simulink model "sampleModel1689"  (R2023a)
settings: Solver=VariableStepAuto  StartTime=0.0  StopTime=10.0  RelTol=1e-3
libraries: hdlsllib x4, simulink x3
settings Model: Creator=user1  LastModifiedBy=user1

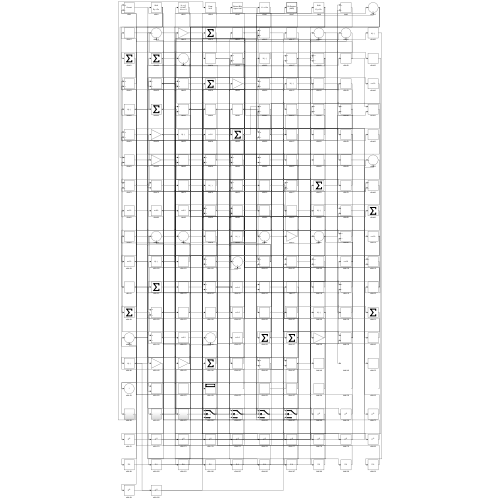
[thumbnail: Simulink's stored preview of the top-level diagram]
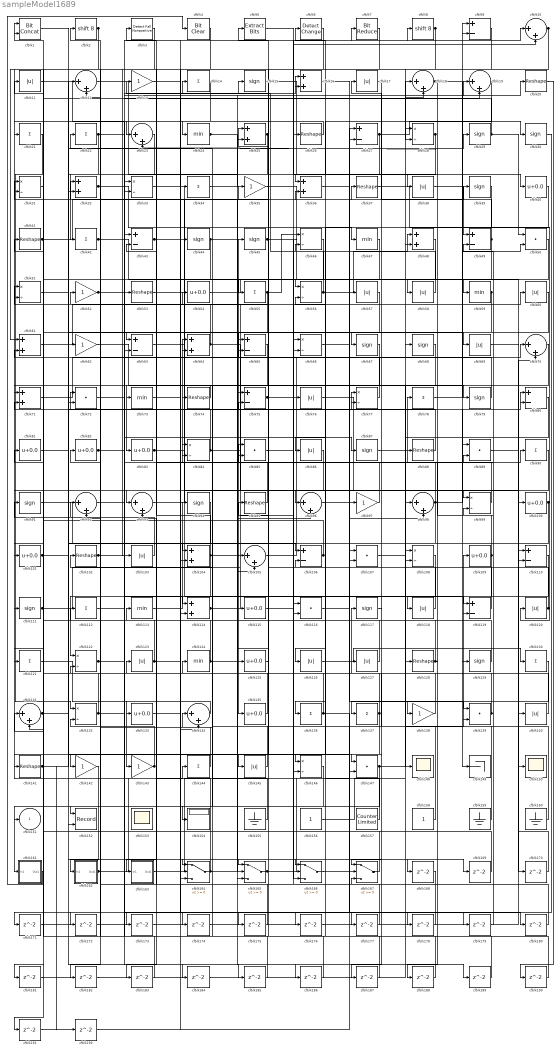
== system sampleModel1689 ==
  cfblk1 : hdlsllib/Logic and Bit Operations/Bit Concat  numInputs=2
  cfblk{10,12,18..19,23,70,92..93,96,98,105,131,134} (13 alike) : Sum  Inputs=|++
  cfblk{40,54,81..83,100..101,109,115,125,133,135} (12 alike) : Bias  Bias=0.0  SaturateOnIntegerOverflow=off
  cfblk{20,26,37,41,53,74,88,95,102,128,141} (11 alike) : Reshape
  cfblk{11,17,38,57..58,60,69,76,86,103,118,120,123,126..127,140,145} (17 alike) : Abs  SaturateOnIntegerOverflow=off
  cfblk{16,25,32,36,48,61,64,71,104,114} (10 alike) : Sum
  cfblk{9,27,43,49,63,65,75,80,106,110,119} (11 alike) : Sum  Inputs=+-
  cfblk{50,72,85,89,107,116,139,147} (8 alike) : DotProduct  OutDataTypeStr=Inherit: Inherit via internal rule
  cfblk{28,31,33,46,51,56,66,77,84,99,108,122,132,146} (14 alike) : Product  Inputs=*/  RndMeth=Zero  SaturateOnIntegerOverflow=on
  cfblk{15,29..30,39,44..45,67..68,79,87,91,94,111,117,129} (15 alike) : Signum
  cfblk{14,21..22,34,42,55,78,90,112,121,130,136..137,144} (14 alike) : Sum  Inputs=+
  cfblk{24,47,59,73,113,124} (6 alike) : MinMax
  cfblk{13,35,52,62,97,138,142..143} (8 alike) : Gain
  cfblk148 : Scope
  cfblk149 : Terminator
  cfblk150 : Scope
  cfblk152 : Record  FileSettingsInternal="{\"entries\":[{\"content\":{\"excelSettings\":{\"content\":{},\"type\":\"Streamout.ExcelSettings\"}},\"type\":\"Streamout.FileSettingStorage\",\"uuid\":\"\"}],\"packageUris\":[\"http:\\/\\/schema.mathworks.com\\/mf0\\/streamout_blocks\\/R2020a\"],\"version\":\"1.0\"}"  Layout=[1 1]  SignalsInternal="{\"entries\":[{\"content\":{\"signals\":[{\"content\":{\"blockPath\":[],\"dimensions\":[1],\"domain\":\"\",\"lineColor\":\"#a2142f\",\"plots\":[1],\"port\":1,\"signalID\":2972,\"signalName\":\"XY Graph:1\"},\"type\":\"RecordBlkView.Signal\",\"uuid\":\"\"},{\"content\":{\"blockPath\":[],\"dimensions\":[1],\"domain\":\"\",\"lineColor\":\"#139fff\",\"plots\":[1],\"port\":2,\"signalID\":2975,\"signalName\":\"XY Graph:2\"},\"type\":\"RecordBlkView.Signal\",\"uuid\":\"\"}]},\"type\":\"RecordBlkView.InputSignals\",\"uuid\":\"\"}],\"packageUris\":[\"http:\\/\\/schema.mathworks.com\\/mf0\\/streamout_blocks\\/R2020a\"],\"version\":\"1.0\"}"  VisualizationBindings="{\"xyplotplugin\":{\"info\":[{\"series\":[{\"bindingParametersList\":[{\"parameter\":\"X-Axis\",\"signalID\":2972,\"signalName\":\"XY Graph:1\"},{\"parameter\":\"Y-Axis\",\"signalID\":2975,\"signalName\":\"XY Graph:2\"}],\"seriesID\":48472}],\"subplotID\":1}]}}"  CompatibilityTag=XY  st=-1
  cfblk153 : Scope
      settings: Floating=on
  cfblk154 : Display
  cfblk155 : Ground
  cfblk156 : Constant  SampleTime=-1
  cfblk157 : hdlsllib/Sources/Counter Limited  uplimit=7  tsamp=-1
  cfblk158 : Constant  SampleTime=-1
  cfblk159 : Ground
  cfblk160 : Ground
  cfblk161 : Subsystem
      settings: LibrarySourceBlock=|
      | hdlsllib/Ports &
      | Subsystems/Subsystem
  cfblk162 : Subsystem
      settings: LibrarySourceBlock=|
      | hdlsllib/Ports &
      | Subsystems/Subsystem
  cfblk163 : Subsystem
      settings: LibrarySourceBlock=|
      | hdlsllib/Ports &
      | Subsystems/Subsystem
  cfblk{164..167} (4 alike) : Switch  SaturateOnIntegerOverflow=off  InputSameDT=off
  cfblk{168..192} (25 alike) : Delay  SampleTime=1
  cfblk2 : ArithShift  BitShiftNumber=8
  cfblk3 : hdlsllib/Logic and Bit Operations/Detect Fall Nonpositive  vinit=0  OutDataTypeStr=boolean
  cfblk4 : simulink/Logic and Bit Operations/Bit Clear  iBit=0
      settings: LibrarySourceBlock=|
      | hdlsllib/Logic and Bit
      | Operations/Bit Clear
  cfblk5 : simulink/Logic and Bit Operations/Extract Bits  bitsToExtract=Upper half  numBits=8  bitIdxRange=[0 7]  outScalingMode=Preserve fixed-point scaling
      settings: LibrarySourceBlock=|
      | hdlsllib/Logic and Bit
      | Operations/Extract Bits
  cfblk6 : simulink/Logic and Bit Operations/Detect Change  vinit=0  OutDataTypeStr=boolean
      settings: LibrarySourceBlock=|
      | hdlsllib/Logic and Bit
      | Operations/Detect
      | Change
  cfblk7 : hdlsllib/Logic and Bit Operations/Bit Reduce  mode=AND
  cfblk8 : ArithShift  BitShiftNumber=8
  cfblk151 : Outport  VectorParamsAs1DForOutWhenUnconnected=off
  wires:
  cfblk55/1 -> cfblk63/1, cfblk46/1
  cfblk120/1 -> cfblk35/1, cfblk31/1
  cfblk138/1 -> cfblk117/1
  cfblk9/1 -> cfblk103/1
  cfblk15/1 -> cfblk40/1
  cfblk93/1 -> cfblk77/1
  cfblk145/1 -> cfblk102/1
  cfblk71/1 -> cfblk70/1
  cfblk58/1 -> cfblk14/1
  cfblk122/1 -> cfblk53/1, cfblk77/2
  cfblk114/1 -> cfblk60/1, cfblk166/1, cfblk176/1
  cfblk54/1 -> cfblk56/1
  cfblk166/1 -> cfblk97/1
  cfblk23/1 -> cfblk142/1
  cfblk37/1 -> cfblk120/1
  cfblk21/1 -> cfblk132/1
  cfblk39/1 -> cfblk136/1
  cfblk31/1 -> cfblk144/1
  cfblk38/1 -> cfblk49/1
  cfblk68/1 -> cfblk83/1
  cfblk155/1 -> cfblk134/1
  cfblk77/1 -> cfblk45/1
  cfblk118/1 -> cfblk51/1
  cfblk33/1 -> cfblk59/1
  cfblk144/1 -> cfblk52/1
  cfblk56/1 -> cfblk48/1, cfblk46/2
  cfblk90/1 -> cfblk111/1
  cfblk2/1 -> cfblk61/1, cfblk32/2, cfblk181/1
  cfblk124/1 -> cfblk113/1, cfblk88/1
  cfblk110/1 -> cfblk122/1
  cfblk91/1 -> cfblk134/2
  cfblk52/1 -> cfblk43/1, cfblk164/1
  cfblk159/1 -> cfblk109/1
  cfblk26/1 -> cfblk24/1
  cfblk48/1 -> cfblk93/1
  cfblk163/1(Out1) -> cfblk27/2
  cfblk102/1 -> cfblk90/1, cfblk185/1
  cfblk140/1 -> cfblk25/1
  cfblk60/1 -> cfblk135/1
  cfblk8/1 -> cfblk23/1, cfblk183/1
  cfblk97/1 -> cfblk6/1
  cfblk121/1 -> cfblk143/1
  cfblk70/1 -> cfblk126/1
  cfblk141/1 -> cfblk29/1, cfblk192/1
  cfblk14/1 -> cfblk101/1
  cfblk87/1 -> cfblk78/1
  cfblk27/1 -> cfblk30/1, cfblk164/3
  cfblk12/1 -> cfblk115/1
  cfblk103/1 -> cfblk91/1
  cfblk157/1 -> cfblk56/2
  cfblk142/1 -> cfblk162/1(In1)
  cfblk10/1 -> cfblk55/1, cfblk114/2, cfblk28/2
  cfblk136/1 -> cfblk82/1, cfblk179/1
  cfblk125/1 -> cfblk95/1
  cfblk127/1 -> cfblk15/1
  cfblk147/1 -> cfblk152/1, cfblk139/2
  cfblk162/1(Out1) -> cfblk34/1, cfblk19/2
  cfblk83/1 -> cfblk9/1, cfblk10/1
  cfblk61/1 -> cfblk9/2
  cfblk158/1 -> cfblk22/1
  cfblk146/1 -> cfblk161/1(In1)
  cfblk53/1 -> cfblk99/1
  cfblk18/1 -> cfblk89/1, cfblk58/1
  cfblk135/1 -> cfblk124/1
  cfblk123/1 -> cfblk39/1, cfblk11/1
  cfblk99/1 -> cfblk64/1
  cfblk49/1 -> cfblk17/1, cfblk165/2, cfblk147/1
  cfblk63/1 -> cfblk119/1
  cfblk43/1 -> cfblk149/1, cfblk76/1, cfblk16/2, cfblk166/2
  cfblk112/1 -> cfblk20/1
  cfblk95/1 -> cfblk3/1
  cfblk29/1 -> cfblk50/1, cfblk1/1
  cfblk74/1 -> cfblk71/1
  cfblk101/1 -> cfblk62/1, cfblk189/1
  cfblk161/1(Out1) -> cfblk4/1
  cfblk113/1 -> cfblk94/1
  cfblk107/1 -> cfblk98/1
  cfblk41/1 -> cfblk37/1, cfblk147/2
  cfblk45/1 -> cfblk150/1, cfblk105/1, cfblk169/1
  cfblk143/1 -> cfblk92/1, cfblk112/1
  cfblk67/1 -> cfblk154/1
  cfblk108/1 -> cfblk146/1
  cfblk5/1 -> cfblk38/1
  cfblk79/1 -> cfblk51/2
  cfblk64/1 -> cfblk116/2, cfblk31/2
  cfblk164/1 -> cfblk123/1, cfblk36/2, cfblk186/1
  cfblk94/1 -> cfblk152/2
  cfblk126/1 -> cfblk130/1
  cfblk119/1 -> cfblk13/1
  cfblk75/1 -> cfblk125/1, cfblk80/2
  cfblk6/1 -> cfblk73/1
  cfblk104/1 -> cfblk61/2, cfblk10/2, cfblk182/1
  cfblk16/1 -> cfblk139/1
  cfblk139/1 -> cfblk119/2, cfblk89/2
  cfblk92/1 -> cfblk7/1
  cfblk130/1 -> cfblk137/1
  cfblk51/1 -> cfblk67/1
  cfblk76/1 -> cfblk140/1
  cfblk116/1 -> cfblk138/1
  cfblk62/1 -> cfblk128/1
  cfblk32/1 -> cfblk65/1, cfblk16/1, cfblk165/3, cfblk174/1
  cfblk115/1 -> cfblk66/1
  cfblk85/1 -> cfblk26/1
  cfblk165/1 -> cfblk57/1, cfblk168/1
  cfblk80/1 -> cfblk108/2
  cfblk24/1 -> cfblk47/1, cfblk66/2
  cfblk57/1 -> cfblk151/1
  cfblk160/1 -> cfblk127/1
  cfblk66/1 -> cfblk107/1
  cfblk109/1 -> cfblk49/2, cfblk146/2, cfblk85/2
  cfblk96/1 -> cfblk98/2
  cfblk134/1 -> cfblk133/1
  cfblk84/1 -> cfblk148/1, cfblk41/1
  cfblk129/1 -> cfblk72/1
  cfblk86/1 -> cfblk121/1
  cfblk11/1 -> cfblk33/2
  cfblk65/1 -> cfblk75/1
  cfblk117/1 -> cfblk167/1
  cfblk22/1 -> cfblk72/2, cfblk104/1
  cfblk72/1 -> cfblk75/2
  cfblk34/1 -> cfblk19/1
  cfblk19/1 -> cfblk36/1
  cfblk59/1 -> cfblk69/1, cfblk145/1
  cfblk105/1 -> cfblk18/2
  cfblk35/1 -> cfblk110/2
  cfblk98/1 -> cfblk163/1(In1), cfblk80/1, cfblk43/2, cfblk166/3
  cfblk47/1 -> cfblk86/1
  cfblk42/1 -> cfblk2/1, cfblk129/1
  cfblk25/1 -> cfblk5/1, cfblk63/2
  cfblk81/1 -> cfblk12/1
  cfblk28/1 -> cfblk42/1, cfblk23/2
  cfblk46/1 -> cfblk65/2
  cfblk40/1 -> cfblk96/1
  cfblk128/1 -> cfblk12/2, cfblk188/1
  cfblk44/1 -> cfblk96/2, cfblk141/1, cfblk105/2
  cfblk106/1 -> cfblk84/1, cfblk71/2
  cfblk132/1 -> cfblk54/1, cfblk81/1
  cfblk82/1 -> cfblk114/1, cfblk87/1
  cfblk7/1 -> cfblk21/1
  cfblk36/1 -> cfblk79/1
  cfblk88/1 -> cfblk32/1
  cfblk78/1 -> cfblk50/2
  cfblk137/1 -> cfblk85/1, cfblk191/1
  cfblk167/1 -> cfblk131/2
  cfblk156/1 -> cfblk68/1
  cfblk69/1 -> cfblk100/1
  cfblk1/1 -> cfblk106/1
  cfblk100/1 -> cfblk118/1, cfblk104/2
  cfblk131/1 -> cfblk165/1, cfblk74/1
  cfblk111/1 -> cfblk8/1, cfblk184/1
  cfblk168/1 -> cfblk167/3
  cfblk169/1 -> cfblk1/2
  cfblk89/1 -> cfblk170/1
  cfblk170/1 -> cfblk110/1
  cfblk30/1 -> cfblk171/1
  cfblk171/1 -> cfblk27/1
  cfblk3/1 -> cfblk172/1
  cfblk172/1 -> cfblk18/1
  cfblk4/1 -> cfblk173/1
  cfblk173/1 -> cfblk108/1
  cfblk174/1 -> cfblk70/2
  cfblk13/1 -> cfblk175/1
  cfblk175/1 -> cfblk132/2
  cfblk176/1 -> cfblk48/2
  cfblk73/1 -> cfblk177/1
  cfblk177/1 -> cfblk93/2
  cfblk50/1 -> cfblk178/1
  cfblk178/1 -> cfblk116/1
  cfblk179/1 -> cfblk99/2
  cfblk133/1 -> cfblk180/1
  cfblk180/1 -> cfblk92/2
  cfblk181/1 -> cfblk28/1
  cfblk182/1 -> cfblk164/2
  cfblk183/1 -> cfblk33/1
  cfblk184/1 -> cfblk107/2
  cfblk185/1 -> cfblk64/2
  cfblk186/1 -> cfblk84/2
  cfblk17/1 -> cfblk187/1
  cfblk187/1 -> cfblk25/2
  cfblk188/1 -> cfblk106/2
  cfblk189/1 -> cfblk122/2
  cfblk20/1 -> cfblk190/1
  cfblk190/1 -> cfblk131/1
  cfblk191/1 -> cfblk167/2
  cfblk192/1 -> cfblk44/1

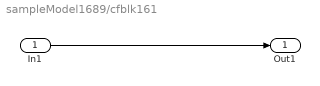
== system sampleModel1689/cfblk161 ==
  In1 : Inport
  Out1 : Outport
  wires:
  In1/1 -> Out1/1

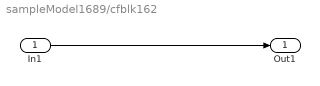
== system sampleModel1689/cfblk162 ==
  In1 : Inport
  Out1 : Outport
  wires:
  In1/1 -> Out1/1

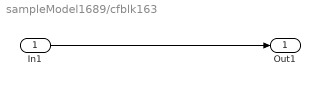
== system sampleModel1689/cfblk163 ==
  In1 : Inport
  Out1 : Outport
  wires:
  In1/1 -> Out1/1
